simulink model "Aerosonde_modeling_3DOF"  (R2023b)
settings: Solver=VariableStepAuto  StartTime=0.0  StopTime=100  RelTol=1e-3
InitFcn:
  | aerosonde_param
model workspace (MAT data in the model file):
  op_trim1 = opcond.OperatingReport
  op_trim1.Outputs_ = opcond.OutputReport
  op_trim1.Outputs_.yspec_ = 23
  op_trim1.Outputs_.Block_ = 'Aerosonde_modeling_3DOF/Va'
  op_trim1.Outputs_.PortWidth_ = 1
  op_trim1.Outputs_.PortNumber_ = NaN
  op_trim1.Outputs_.y_ = 23
  op_trim1.Outputs_.Known_ = 1
  op_trim1.Outputs_.Min_ = -Inf
  op_trim1.Outputs_.Max_ = Inf
  op_trim1.TerminationString_ = 'Operating point specifications were successfully met.'
  op_trim1.OptimizationOutput_.iterations = 4
  op_trim1.OptimizationOutput_.funcCount = 49
  op_trim1.OptimizationOutput_.lssteplength = 1
  op_trim1.OptimizationOutput_.stepsize = 1.08339920389e-06
  op_trim1.OptimizationOutput_.algorithm = 'active-set'
  op_trim1.OptimizationOutput_.firstorderopt = 6.92917038473e-07
  op_trim1.OptimizationOutput_.constrviolation = 4.1486832541e-10
  op_trim1.OptimizationOutput_.message = 'Local minimum found that satisfies the constraints.
    | 
    | Optimization completed because the objective function is non-decreasing in 
    | feasible directions, to within the value of the optimality tolerance,
    | and constraints are satisfied to within the  value of the constraint tolerance.
    | 
    | <stopping criteria details>
    | 
    | Optimization completed: The first-order optimality measure, 6.929170e-07, is less
    | than options.OptimalityTolerance = 1.000000e-06, and the maximum constraint violation,
    | 4.148683e-10,is less than options.ConstraintTolerance = 1.000000e-06.'
  op_trim1.OptimizationOutput_.bestfeasible.x = [22.8390288243; 2.71638774139; 3.14319268182e-07; -200.000000001; -2.24898193262e-22; 0.11838011473; -0.136728887195; 0.391911265794]
  op_trim1.OptimizationOutput_.bestfeasible.fval = 0
  op_trim1.OptimizationOutput_.bestfeasible.constrviolation = 4.1486832541e-10
  op_trim1.OptimizationOutput_.bestfeasible.firstorderopt = 6.92917038473e-07
  op_trim1.OptimizationOutput_.progress = {'<font face="monospaced"; size=3><BR>', 'Optimizing to solve for all desired dx/dt=0, x(k+1)-x(k)=0, and y=ydes.<BR>', ' <BR>', '(Maximum Error)  Block<BR>', ' ---------------------------------------------------------<BR>', '(6.14386e+00) Aerosonde_modeling_3DOF/3dof (Body Axes)<BR>', '(7.32692e-01) Aerosonde_modeling_3DOF/3dof (Body Axes)<BR>', '(7.37961e-04) Aerosonde_modeling_3DOF/3dof (Body Axes)<BR>', '(2.36211e-06) Aerosonde_modeling_3DOF/3dof (Body Axes)<BR>', '(4.14856e-10) Aerosonde_modeling_3DOF/3dof (Body Axes)<BR>', '(4.14856e-10) Aerosonde_modeling_3DOF/3dof (Body Axes)<BR>', ' <BR>', 'Operating point specifications were successfully met.<BR>'}
  op_trim1.Model_ = 'Aerosonde_modeling_3DOF'
  op_trim1.States_(1) = opcond.StateReport
  op_trim1.States_(1).dx_ = 6.55270405843e-11
  op_trim1.States_(1).Nx_ = 1
  op_trim1.States_(1).Block_ = 'Aerosonde_modeling_3DOF/3dof (Body Axes)'
  op_trim1.States_(1).StateName_ = 'u'
  op_trim1.States_(1).x_ = 22.8390288243
  op_trim1.States_(1).SteadyState_ = 1
  op_trim1.States_(1).dxMin_ = -Inf
  op_trim1.States_(1).dxMax_ = Inf
  op_trim1.States_(1).Known_ = 0
  op_trim1.States_(1).Min_ = -Inf
  op_trim1.States_(1).Max_ = Inf
  op_trim1.States_(2) = opcond.StateReport
  op_trim1.States_(2).dx_ = -4.14855902722e-10
  op_trim1.States_(2).Nx_ = 1
  op_trim1.States_(2).Block_ = 'Aerosonde_modeling_3DOF/3dof (Body Axes)'
  op_trim1.States_(2).StateName_ = 'w'
  op_trim1.States_(2).x_ = 2.71638774139
  op_trim1.States_(2).SteadyState_ = 1
  op_trim1.States_(2).dxMin_ = -Inf
  op_trim1.States_(2).dxMax_ = Inf
  op_trim1.States_(2).Known_ = 0
  op_trim1.States_(2).Min_ = -Inf
  op_trim1.States_(2).Max_ = Inf
  op_trim1.States_(3) = opcond.StateReport
  op_trim1.States_(3).dx_ = 23
  op_trim1.States_(3).Nx_ = 1
  op_trim1.States_(3).Block_ = 'Aerosonde_modeling_3DOF/3dof (Body Axes)'
  op_trim1.States_(3).StateName_ = 'Xe'
  op_trim1.States_(3).x_ = 3.14319268182e-07
  op_trim1.States_(3).SteadyState_ = 0
  op_trim1.States_(3).dxMin_ = -Inf
  op_trim1.States_(3).dxMax_ = Inf
  op_trim1.States_(3).Known_ = 0
  op_trim1.States_(3).Min_ = -Inf
  op_trim1.States_(3).Max_ = Inf
  op_trim1.States_(4) = opcond.StateReport
  op_trim1.States_(4).dx_ = 8.881784197e-16
  op_trim1.States_(4).Nx_ = 1
  op_trim1.States_(4).Block_ = 'Aerosonde_modeling_3DOF/3dof (Body Axes)'
  op_trim1.States_(4).StateName_ = 'Ze'
  op_trim1.States_(4).x_ = -200.000000001
  op_trim1.States_(4).SteadyState_ = 1
  op_trim1.States_(4).dxMin_ = -Inf
  op_trim1.States_(4).dxMax_ = Inf
  op_trim1.States_(4).Known_ = 0
  op_trim1.States_(4).Min_ = -Inf
  op_trim1.States_(4).Max_ = Inf
  op_trim1.States_(5) = opcond.StateReport
  op_trim1.States_(5).dx_ = -1.36577515895e-14
  op_trim1.States_(5).Nx_ = 1
  op_trim1.States_(5).Block_ = 'Aerosonde_modeling_3DOF/3dof (Body Axes)'
  op_trim1.States_(5).StateName_ = 'q'
  op_trim1.States_(5).x_ = -2.24898193262e-22
  op_trim1.States_(5).SteadyState_ = 1
  op_trim1.States_(5).dxMin_ = -Inf
  op_trim1.States_(5).dxMax_ = Inf
  op_trim1.States_(5).Known_ = 0
  op_trim1.States_(5).Min_ = -Inf
  op_trim1.States_(5).Max_ = Inf
  op_trim1.States_(6) = opcond.StateReport
  op_trim1.States_(6).dx_ = -2.24898193262e-22
  op_trim1.States_(6).Nx_ = 1
  op_trim1.States_(6).Block_ = 'Aerosonde_modeling_3DOF/3dof (Body Axes)'
  op_trim1.States_(6).StateName_ = 'theta'
  op_trim1.States_(6).x_ = 0.11838011473
  op_trim1.States_(6).SteadyState_ = 1
  op_trim1.States_(6).dxMin_ = -Inf
  op_trim1.States_(6).dxMax_ = Inf
  op_trim1.States_(6).Known_ = 0
  op_trim1.States_(6).Min_ = -Inf
  op_trim1.States_(6).Max_ = Inf
  op_trim1.Inputs_(1) = opcond.InputReport
  op_trim1.Inputs_(1).Block_ = 'Aerosonde_modeling_3DOF/ELE'
  op_trim1.Inputs_(1).PortWidth_ = 1
  op_trim1.Inputs_(1).PortDimensions_ = [1 1]
  op_trim1.Inputs_(1).u_ = -0.136728887195
  op_trim1.Inputs_(1).Known_ = 0
  op_trim1.Inputs_(1).Min_ = -Inf
  op_trim1.Inputs_(1).Max_ = Inf
  op_trim1.Inputs_(2) = opcond.InputReport
  op_trim1.Inputs_(2).Block_ = 'Aerosonde_modeling_3DOF/THR'
  op_trim1.Inputs_(2).PortWidth_ = 1
  op_trim1.Inputs_(2).PortDimensions_ = [1 1]
  op_trim1.Inputs_(2).u_ = 0.391911265794
  op_trim1.Inputs_(2).Known_ = 0
  op_trim1.Inputs_(2).Min_ = 0
  op_trim1.Inputs_(2).Max_ = 1
  op_trim2 = opcond.OperatingReport
  op_trim2.Outputs_ = opcond.OutputReport
  op_trim2.Outputs_.yspec_ = 23
  op_trim2.Outputs_.Block_ = 'Aerosonde_modeling/Va'
  op_trim2.Outputs_.PortWidth_ = 1
  op_trim2.Outputs_.PortNumber_ = NaN
  op_trim2.Outputs_.y_ = 0.022563556599
  op_trim2.Outputs_.Known_ = 1
  op_trim2.Outputs_.Min_ = -Inf
  op_trim2.Outputs_.Max_ = Inf
  op_trim2.TerminationString_ = 'Operating point specifications were successfully met.'
  op_trim2.OptimizationOutput_.iterations = 1
  op_trim2.OptimizationOutput_.funcCount = 10
  op_trim2.OptimizationOutput_.stepsize = 25.3486722495
  op_trim2.OptimizationOutput_.cgiterations = []
  op_trim2.OptimizationOutput_.firstorderopt = 45.6856066461
  op_trim2.OptimizationOutput_.algorithm = 'levenberg-marquardt'
  op_trim2.OptimizationOutput_.message = 'Local minimum possible.
    | lsqnonlin stopped because the relative size of the current step is less than
    | the value of the step size tolerance.
    | 
    | <stopping criteria details>
    | 
    | Optimization stopped because the relative norm of the current step, 2.607750e-07,
    | is less than options.StepTolerance = 1.000000e-06.'
  op_trim2.OptimizationOutput_.bestfeasible = []
  op_trim2.OptimizationOutput_.constrviolation = []
  op_trim2.OptimizationOutput_.progress = {'<font face="monospaced"; size=3><BR>', 'Optimizing to solve for all desired dx/dt=0, x(k+1)-x(k)=0, and y=ydes.<BR>', ' <BR>', '(Maximum Error)  Block<BR>', ' ---------------------------------------------------------<BR>', '(2.29774e+01) Aerosonde_modeling/Va<BR>', '(2.29774e+01) Aerosonde_modeling/Va<BR>', ' <BR>', 'Operating point specifications were successfully met.<BR>'}
  op_trim2.Model_ = 'Aerosonde_modeling'
  op_trim2.States_(1) = opcond.StateReport
  op_trim2.States_(1).dx_ = -11.6769691065
  op_trim2.States_(1).Nx_ = 1
  op_trim2.States_(1).Block_ = 'Aerosonde_modeling/3dof (Body Axes)'
  op_trim2.States_(1).StateName_ = 'u'
  op_trim2.States_(1).x_ = -0.00779019632016
  op_trim2.States_(1).SteadyState_ = 1
  op_trim2.States_(1).dxMin_ = -Inf
  op_trim2.States_(1).dxMax_ = Inf
  op_trim2.States_(1).Known_ = 0
  op_trim2.States_(1).Min_ = -Inf
  op_trim2.States_(1).Max_ = Inf
  op_trim2.States_(2) = opcond.StateReport
  op_trim2.States_(2).dx_ = -15.7183253748
  op_trim2.States_(2).Nx_ = 1
  op_trim2.States_(2).Block_ = 'Aerosonde_modeling/3dof (Body Axes)'
  op_trim2.States_(2).StateName_ = 'w'
  op_trim2.States_(2).x_ = 0.0211760933056
  op_trim2.States_(2).SteadyState_ = 1
  op_trim2.States_(2).dxMin_ = -Inf
  op_trim2.States_(2).dxMax_ = Inf
  op_trim2.States_(2).Known_ = 0
  op_trim2.States_(2).Min_ = -Inf
  op_trim2.States_(2).Max_ = Inf
  op_trim2.States_(3) = opcond.StateReport
  op_trim2.States_(3).dx_ = 0.0188976239913
  op_trim2.States_(3).Nx_ = 1
  op_trim2.States_(3).Block_ = 'Aerosonde_modeling/3dof (Body Axes)'
  op_trim2.States_(3).StateName_ = 'Xe'
  op_trim2.States_(3).x_ = -7461695.80517
  op_trim2.States_(3).SteadyState_ = 0
  op_trim2.States_(3).dxMin_ = -Inf
  op_trim2.States_(3).dxMax_ = Inf
  op_trim2.States_(3).Known_ = 0
  op_trim2.States_(3).Min_ = -Inf
  op_trim2.States_(3).Max_ = Inf
  op_trim2.States_(4) = opcond.StateReport
  op_trim2.States_(4).dx_ = -0.0123285803676
  op_trim2.States_(4).Nx_ = 1
  op_trim2.States_(4).Block_ = 'Aerosonde_modeling/3dof (Body Axes)'
  op_trim2.States_(4).StateName_ = 'Ze'
  op_trim2.States_(4).x_ = 96918353.295
  op_trim2.States_(4).SteadyState_ = 0
  op_trim2.States_(4).dxMin_ = -Inf
  op_trim2.States_(4).dxMax_ = Inf
  op_trim2.States_(4).Known_ = 0
  op_trim2.States_(4).Min_ = -Inf
  op_trim2.States_(4).Max_ = Inf
  op_trim2.States_(5) = opcond.StateReport
  op_trim2.States_(5).dx_ = -0.000422280268139
  op_trim2.States_(5).Nx_ = 1
  op_trim2.States_(5).Block_ = 'Aerosonde_modeling/3dof (Body Axes)'
  op_trim2.States_(5).StateName_ = 'q'
  op_trim2.States_(5).x_ = -2.06010862536
  op_trim2.States_(5).SteadyState_ = 1
  op_trim2.States_(5).dxMin_ = -Inf
  op_trim2.States_(5).dxMax_ = Inf
  op_trim2.States_(5).Known_ = 0
  op_trim2.States_(5).Min_ = -Inf
  op_trim2.States_(5).Max_ = Inf
  op_trim2.States_(6) = opcond.StateReport
  op_trim2.States_(6).dx_ = -2.06010862536
  op_trim2.States_(6).Nx_ = 1
  op_trim2.States_(6).Block_ = 'Aerosonde_modeling/3dof (Body Axes)'
  op_trim2.States_(6).StateName_ = 'theta'
  op_trim2.States_(6).x_ = 2.50135956362
  op_trim2.States_(6).SteadyState_ = 1
  op_trim2.States_(6).dxMin_ = -Inf
  op_trim2.States_(6).dxMax_ = Inf
  op_trim2.States_(6).Known_ = 0
  op_trim2.States_(6).Min_ = -Inf
  op_trim2.States_(6).Max_ = Inf
  op_trim2.Inputs_(1) = opcond.InputReport
  op_trim2.Inputs_(1).Block_ = 'Aerosonde_modeling/ele'
  op_trim2.Inputs_(1).PortWidth_ = 1
  op_trim2.Inputs_(1).PortDimensions_ = [1 1]
  op_trim2.Inputs_(1).u_ = 6.80738411077e-06
  op_trim2.Inputs_(1).Known_ = 0
  op_trim2.Inputs_(1).Min_ = -Inf
  op_trim2.Inputs_(1).Max_ = Inf
  op_trim2.Inputs_(2) = opcond.InputReport
  op_trim2.Inputs_(2).Block_ = 'Aerosonde_modeling/THR'
  op_trim2.Inputs_(2).PortWidth_ = 1
  op_trim2.Inputs_(2).PortDimensions_ = [1 1]
  op_trim2.Inputs_(2).Known_ = 0
  op_trim2.Inputs_(2).Min_ = 0
  op_trim2.Inputs_(2).Max_ = 1
  op_trim5 = opcond.OperatingReport
  op_trim5.Outputs_ = opcond.OutputReport
  op_trim5.Outputs_.yspec_ = [0; 0; 0; 0; 0; 0; 0]
  op_trim5.Outputs_.Block_ = 'Aerosonde_modeling/States'
  op_trim5.Outputs_.PortWidth_ = 7
  op_trim5.Outputs_.PortNumber_ = NaN
  op_trim5.Outputs_.y_ = [-0.614028193896; 9.4193417265e-05; 2.52756048863; -208278.082793; -1.81540582654e-06; -7461695.80517; 96918353.295]
  op_trim5.Outputs_.Known_ = [0; 0; 0; 0; 0; 0; 0]
  op_trim5.Outputs_.Min_ = [-Inf; -Inf; -Inf; -Inf; -Inf; -Inf; -Inf]
  op_trim5.Outputs_.Max_ = [Inf; Inf; Inf; Inf; Inf; Inf; Inf]
  op_trim5.TerminationString_ = 'Maximum number of function evaluations or iterations was exceeded.  Restart using this resulting solution or use the Optimization Options to increase the number of iterations or function evaluations.'
  op_trim5.OptimizationOutput_.iterations = 101
  op_trim5.OptimizationOutput_.funcCount = 2007
  op_trim5.OptimizationOutput_.lssteplength = 1
  op_trim5.OptimizationOutput_.stepsize = 136552843.933
  op_trim5.OptimizationOutput_.algorithm = 'active-set'
  op_trim5.OptimizationOutput_.firstorderopt = 3.30032720888e+32
  op_trim5.OptimizationOutput_.constrviolation = 15.4518372632
  op_trim5.OptimizationOutput_.message = 'Solver stopped prematurely.
    | 
    | fmincon stopped because it exceeded the function evaluation limit,
    | options.MaxFunctionEvaluations = 2.000000e+03.'
  op_trim5.OptimizationOutput_.bestfeasible = []
  op_trim5.OptimizationOutput_.progress{1} = '<font face="monospaced"; size=3><BR>'
  op_trim5.OptimizationOutput_.progress{2} = 'Optimizing to solve for all desired dx/dt=0, x(k+1)-x(k)=0, and y=ydes.<BR>'
  op_trim5.OptimizationOutput_.progress{3} = ' <BR>'
  op_trim5.OptimizationOutput_.progress{4} = '(Maximum Error)  Block<BR>'
  op_trim5.OptimizationOutput_.progress{5} = ' ---------------------------------------------------------<BR>'
  op_trim5.OptimizationOutput_.progress{6} = '(1.59239e+01) Aerosonde_modeling/3dof (Body Axes)<BR>'
  op_trim5.OptimizationOutput_.progress{7} = '(1.21166e+01) Aerosonde_modeling/3dof (Body Axes)<BR>'
  op_trim5.OptimizationOutput_.progress{8} = '(1.38079e+01) Aerosonde_modeling/3dof (Body Axes)<BR>'
  op_trim5.OptimizationOutput_.progress{9} = '(1.13106e+01) Aerosonde_modeling/3dof (Body Axes)<BR>'
  op_trim5.OptimizationOutput_.progress{10} = '(1.02919e+01) Aerosonde_modeling/3dof (Body Axes)<BR>'
  op_trim5.OptimizationOutput_.progress{11} = '(1.01299e+01) Aerosonde_modeling/3dof (Body Axes)<BR>'
  op_trim5.OptimizationOutput_.progress{12} = '(9.17454e+00) Aerosonde_modeling/3dof (Body Axes)<BR>'
  op_trim5.OptimizationOutput_.progress{13} = '(9.40157e+00) Aerosonde_modeling/3dof (Body Axes)<BR>'
  op_trim5.OptimizationOutput_.progress{14} = '(9.38043e+00) Aerosonde_modeling/3dof (Body Axes)<BR>'
  op_trim5.OptimizationOutput_.progress{15} = '(2.10526e+01) Aerosonde_modeling/3dof (Body Axes)<BR>'
  op_trim5.OptimizationOutput_.progress{16} = '(3.47072e+00) Aerosonde_modeling/3dof (Body Axes)<BR>'
  op_trim5.OptimizationOutput_.progress{17} = '(3.78939e+00) Aerosonde_modeling/3dof (Body Axes)<BR>'
  op_trim5.OptimizationOutput_.progress{18} = '(3.98713e+00) Aerosonde_modeling/3dof (Body Axes)<BR>'
  op_trim5.OptimizationOutput_.progress{19} = '(4.10860e+00) Aerosonde_modeling/3dof (Body Axes)<BR>'
  op_trim5.OptimizationOutput_.progress{20} = '(4.18159e+00) Aerosonde_modeling/3dof (Body Axes)<BR>'
  op_trim5.OptimizationOutput_.progress{21} = '(4.22397e+00) Aerosonde_modeling/3dof (Body Axes)<BR>'
  op_trim5.OptimizationOutput_.progress{22} = '(4.24743e+00) Aerosonde_modeling/3dof (Body Axes)<BR>'
  op_trim5.OptimizationOutput_.progress{23} = '(4.25987e+00) Aerosonde_modeling/3dof (Body Axes)<BR>'
  op_trim5.OptimizationOutput_.progress{24} = '(4.26683e+00) Aerosonde_modeling/3dof (Body Axes)<BR>'
  op_trim5.OptimizationOutput_.progress{25} = '(4.27250e+00) Aerosonde_modeling/3dof (Body Axes)<BR>'
  op_trim5.OptimizationOutput_.progress{26} = '(4.28040e+00) Aerosonde_modeling/3dof (Body Axes)<BR>'
  op_trim5.OptimizationOutput_.progress{27} = '(4.01629e+00) Aerosonde_modeling/3dof (Body Axes)<BR>'
  op_trim5.OptimizationOutput_.progress{28} = '(3.78539e+00) Aerosonde_modeling/3dof (Body Axes)<BR>'
  op_trim5.OptimizationOutput_.progress{29} = '(3.57876e+00) Aerosonde_modeling/3dof (Body Axes)<BR>'
  op_trim5.OptimizationOutput_.progress{30} = '(3.39552e+00) Aerosonde_modeling/3dof (Body Axes)<BR>'
  op_trim5.OptimizationOutput_.progress{31} = '(3.22558e+00) Aerosonde_modeling/3dof (Body Axes)<BR>'
  op_trim5.OptimizationOutput_.progress{32} = '(3.03135e+00) Aerosonde_modeling/3dof (Body Axes)<BR>'
  op_trim5.OptimizationOutput_.progress{33} = '(2.87139e+00) Aerosonde_modeling/3dof (Body Axes)<BR>'
  op_trim5.OptimizationOutput_.progress{34} = '(2.84211e+00) Aerosonde_modeling/3dof (Body Axes)<BR>'
  op_trim5.OptimizationOutput_.progress{35} = '(2.82876e+00) Aerosonde_modeling/3dof (Body Axes)<BR>'
  op_trim5.OptimizationOutput_.progress{36} = '(2.90329e+00) Aerosonde_modeling/3dof (Body Axes)<BR>'
  op_trim5.OptimizationOutput_.progress{37} = '(2.90505e+00) Aerosonde_modeling/3dof (Body Axes)<BR>'
  op_trim5.OptimizationOutput_.progress{38} = '(2.90504e+00) Aerosonde_modeling/3dof (Body Axes)<BR>'
  op_trim5.OptimizationOutput_.progress{39} = '(2.90550e+00) Aerosonde_modeling/3dof (Body Axes)<BR>'
  op_trim5.OptimizationOutput_.progress{40} = '(2.90559e+00) Aerosonde_modeling/3dof (Body Axes)<BR>'
  op_trim5.OptimizationOutput_.progress{41} = '(2.90559e+00) Aerosonde_modeling/3dof (Body Axes)<BR>'
  op_trim5.OptimizationOutput_.progress{42} = '(2.90564e+00) Aerosonde_modeling/3dof (Body Axes)<BR>'
  op_trim5.OptimizationOutput_.progress{43} = '(2.90590e+00) Aerosonde_modeling/3dof (Body Axes)<BR>'
  op_trim5.OptimizationOutput_.progress{44} = '(2.90602e+00) Aerosonde_modeling/3dof (Body Axes)<BR>'
  op_trim5.OptimizationOutput_.progress{45} = '(2.90602e+00) Aerosonde_modeling/3dof (Body Axes)<BR>'
  op_trim5.OptimizationOutput_.progress{46} = '(2.90602e+00) Aerosonde_modeling/3dof (Body Axes)<BR>'
  op_trim5.OptimizationOutput_.progress{47} = '(2.90602e+00) Aerosonde_modeling/3dof (Body Axes)<BR>'
  op_trim5.OptimizationOutput_.progress{48} = '(2.90602e+00) Aerosonde_modeling/3dof (Body Axes)<BR>'
  op_trim5.OptimizationOutput_.progress{49} = '(2.90602e+00) Aerosonde_modeling/3dof (Body Axes)<BR>'
  op_trim5.OptimizationOutput_.progress{50} = '(2.90602e+00) Aerosonde_modeling/3dof (Body Axes)<BR>'
  op_trim5.OptimizationOutput_.progress{51} = '(2.90602e+00) Aerosonde_modeling/3dof (Body Axes)<BR>'
  op_trim5.OptimizationOutput_.progress{52} = '(2.90602e+00) Aerosonde_modeling/3dof (Body Axes)<BR>'
  op_trim5.OptimizationOutput_.progress{53} = '(2.90602e+00) Aerosonde_modeling/3dof (Body Axes)<BR>'
  op_trim5.OptimizationOutput_.progress{54} = '(2.90602e+00) Aerosonde_modeling/3dof (Body Axes)<BR>'
  op_trim5.OptimizationOutput_.progress{55} = '(2.90602e+00) Aerosonde_modeling/3dof (Body Axes)<BR>'
  op_trim5.OptimizationOutput_.progress{56} = '(2.90602e+00) Aerosonde_modeling/3dof (Body Axes)<BR>'
  op_trim5.OptimizationOutput_.progress{57} = '(2.90602e+00) Aerosonde_modeling/3dof (Body Axes)<BR>'
  op_trim5.OptimizationOutput_.progress{58} = '(2.90602e+00) Aerosonde_modeling/3dof (Body Axes)<BR>'
  op_trim5.OptimizationOutput_.progress{59} = '(2.90602e+00) Aerosonde_modeling/3dof (Body Axes)<BR>'
  op_trim5.OptimizationOutput_.progress{60} = '(2.90602e+00) Aerosonde_modeling/3dof (Body Axes)<BR>'
  op_trim5.OptimizationOutput_.progress{61} = '(2.90602e+00) Aerosonde_modeling/3dof (Body Axes)<BR>'
  op_trim5.OptimizationOutput_.progress{62} = '(2.90602e+00) Aerosonde_modeling/3dof (Body Axes)<BR>'
  op_trim5.OptimizationOutput_.progress{63} = '(2.90602e+00) Aerosonde_modeling/3dof (Body Axes)<BR>'
  op_trim5.OptimizationOutput_.progress{64} = '(2.90602e+00) Aerosonde_modeling/3dof (Body Axes)<BR>'
  op_trim5.OptimizationOutput_.progress{65} = '(2.90602e+00) Aerosonde_modeling/3dof (Body Axes)<BR>'
  op_trim5.OptimizationOutput_.progress{66} = '(2.90602e+00) Aerosonde_modeling/3dof (Body Axes)<BR>'
  op_trim5.OptimizationOutput_.progress{67} = '(2.90602e+00) Aerosonde_modeling/3dof (Body Axes)<BR>'
  op_trim5.OptimizationOutput_.progress{68} = '(2.90602e+00) Aerosonde_modeling/3dof (Body Axes)<BR>'
  op_trim5.OptimizationOutput_.progress{69} = '(2.90602e+00) Aerosonde_modeling/3dof (Body Axes)<BR>'
  op_trim5.OptimizationOutput_.progress{70} = '(2.90602e+00) Aerosonde_modeling/3dof (Body Axes)<BR>'
  op_trim5.OptimizationOutput_.progress{71} = '(2.90602e+00) Aerosonde_modeling/3dof (Body Axes)<BR>'
  op_trim5.OptimizationOutput_.progress{72} = '(2.90606e+00) Aerosonde_modeling/3dof (Body Axes)<BR>'
  op_trim5.OptimizationOutput_.progress{73} = '(2.75093e+00) Aerosonde_modeling/3dof (Body Axes)<BR>'
  op_trim5.OptimizationOutput_.progress{74} = '(3.54582e+00) Aerosonde_modeling/3dof (Body Axes)<BR>'
  op_trim5.OptimizationOutput_.progress{75} = '(3.89297e+00) Aerosonde_modeling/3dof (Body Axes)<BR>'
  op_trim5.OptimizationOutput_.progress{76} = '(4.14986e+00) Aerosonde_modeling/3dof (Body Axes)<BR>'
  op_trim5.OptimizationOutput_.progress{77} = '(3.55999e+00) Aerosonde_modeling/3dof (Body Axes)<BR>'
  op_trim5.OptimizationOutput_.progress{78} = '(3.20494e+00) Aerosonde_modeling/3dof (Body Axes)<BR>'
  op_trim5.OptimizationOutput_.progress{79} = '(3.18668e+00) Aerosonde_modeling/3dof (Body Axes)<BR>'
  op_trim5.OptimizationOutput_.progress{80} = '(3.13765e+00) Aerosonde_modeling/3dof (Body Axes)<BR>'
  op_trim5.OptimizationOutput_.progress{81} = '(2.68545e+00) Aerosonde_modeling/3dof (Body Axes)<BR>'
  op_trim5.OptimizationOutput_.progress{82} = '(1.76493e-01) Aerosonde_modeling/3dof (Body Axes)<BR>'
  op_trim5.OptimizationOutput_.progress{83} = '(2.34829e-01) Aerosonde_modeling/3dof (Body Axes)<BR>'
  op_trim5.OptimizationOutput_.progress{84} = '(2.35613e-01) Aerosonde_modeling/3dof (Body Axes)<BR>'
  op_trim5.OptimizationOutput_.progress{85} = '(2.35160e-01) Aerosonde_modeling/3dof (Body Axes)<BR>'
  op_trim5.OptimizationOutput_.progress{86} = '(2.34644e-01) Aerosonde_modeling/3dof (Body Axes)<BR>'
  op_trim5.OptimizationOutput_.progress{87} = '(2.34133e-01) Aerosonde_modeling/3dof (Body Axes)<BR>'
  op_trim5.OptimizationOutput_.progress{88} = '(2.33579e-01) Aerosonde_modeling/3dof (Body Axes)<BR>'
  op_trim5.OptimizationOutput_.progress{89} = '(2.33121e-01) Aerosonde_modeling/3dof (Body Axes)<BR>'
  op_trim5.OptimizationOutput_.progress{90} = '(2.33001e-01) Aerosonde_modeling/3dof (Body Axes)<BR>'
  op_trim5.OptimizationOutput_.progress{91} = '(2.32485e-01) Aerosonde_modeling/3dof (Body Axes)<BR>'
  op_trim5.OptimizationOutput_.progress{92} = '(2.31943e-01) Aerosonde_modeling/3dof (Body Axes)<BR>'
  op_trim5.OptimizationOutput_.progress{93} = '(2.31688e-01) Aerosonde_modeling/3dof (Body Axes)<BR>'
  op_trim5.OptimizationOutput_.progress{94} = '(2.31184e-01) Aerosonde_modeling/3dof (Body Axes)<BR>'
  op_trim5.OptimizationOutput_.progress{95} = '(2.30618e-01) Aerosonde_modeling/3dof (Body Axes)<BR>'
  op_trim5.OptimizationOutput_.progress{96} = '(2.44391e-02) Aerosonde_modeling/3dof (Body Axes)<BR>'
  op_trim5.OptimizationOutput_.progress{97} = '(4.66230e-02) Aerosonde_modeling/3dof (Body Axes)<BR>'
  op_trim5.OptimizationOutput_.progress{98} = '(2.92160e-03) Aerosonde_modeling/3dof (Body Axes)<BR>'
  op_trim5.OptimizationOutput_.progress{99} = '(1.24310e-03) Aerosonde_modeling/3dof (Body Axes)<BR>'
  op_trim5.OptimizationOutput_.progress{100} = '(1.24307e-03) Aerosonde_modeling/3dof (Body Axes)<BR>'
  op_trim5.OptimizationOutput_.progress{101} = '(1.24305e-03) Aerosonde_modeling/3dof (Body Axes)<BR>'
  op_trim5.OptimizationOutput_.progress{102} = '(1.24303e-03) Aerosonde_modeling/3dof (Body Axes)<BR>'
  op_trim5.OptimizationOutput_.progress{103} = '(1.24300e-03) Aerosonde_modeling/3dof (Body Axes)<BR>'
  op_trim5.OptimizationOutput_.progress{104} = '(1.24298e-03) Aerosonde_modeling/3dof (Body Axes)<BR>'
  op_trim5.OptimizationOutput_.progress{105} = '(1.24296e-03) Aerosonde_modeling/3dof (Body Axes)<BR>'
  op_trim5.OptimizationOutput_.progress{106} = '(1.24293e-03) Aerosonde_modeling/3dof (Body Axes)<BR>'
  op_trim5.OptimizationOutput_.progress{107} = '(1.54518e+01) Aerosonde_modeling/3dof (Body Axes)<BR>'
  op_trim5.OptimizationOutput_.progress{108} = '(1.24293e-03) Aerosonde_modeling/3dof (Body Axes)<BR>'
  op_trim5.OptimizationOutput_.progress{109} = ' <BR>'
  op_trim5.OptimizationOutput_.progress{110} = 'Maximum number of function evaluations or iterations was exceeded.  Restart using this resulting solution or use the Optimization Options to increase the number of iterations or function evaluations.<BR>'
  op_trim5.Model_ = 'Aerosonde_modeling'
  op_trim5.States_(1) = opcond.StateReport
  op_trim5.States_(1).dx_ = -0.00097150794859
  op_trim5.States_(1).Nx_ = 1
  op_trim5.States_(1).Block_ = 'Aerosonde_modeling/3dof (Body Axes)'
  op_trim5.States_(1).StateName_ = 'u'
  op_trim5.States_(1).x_ = -7.69874592357e-05
  op_trim5.States_(1).SteadyState_ = 1
  op_trim5.States_(1).dxMin_ = -Inf
  op_trim5.States_(1).dxMax_ = Inf
  op_trim5.States_(1).Known_ = 0
  op_trim5.States_(1).Min_ = -Inf
  op_trim5.States_(1).Max_ = Inf
  op_trim5.States_(2) = opcond.StateReport
  op_trim5.States_(2).dx_ = -0.00124293328653
  op_trim5.States_(2).Nx_ = 1
  op_trim5.States_(2).Block_ = 'Aerosonde_modeling/3dof (Body Axes)'
  op_trim5.States_(2).StateName_ = 'w'
  op_trim5.States_(2).x_ = 5.42709035901e-05
  op_trim5.States_(2).SteadyState_ = 1
  op_trim5.States_(2).dxMin_ = -Inf
  op_trim5.States_(2).dxMax_ = Inf
  op_trim5.States_(2).Known_ = 0
  op_trim5.States_(2).Min_ = -Inf
  op_trim5.States_(2).Max_ = Inf
  op_trim5.States_(3) = opcond.StateReport
  op_trim5.States_(3).dx_ = 9.41934172643e-05
  op_trim5.States_(3).Nx_ = 1
  op_trim5.States_(3).Block_ = 'Aerosonde_modeling/3dof (Body Axes)'
  op_trim5.States_(3).StateName_ = 'Xe'
  op_trim5.States_(3).x_ = -7461695.80517
  op_trim5.States_(3).SteadyState_ = 0
  op_trim5.States_(3).dxMin_ = -Inf
  op_trim5.States_(3).dxMax_ = Inf
  op_trim5.States_(3).Known_ = 0
  op_trim5.States_(3).Min_ = -Inf
  op_trim5.States_(3).Max_ = Inf
  op_trim5.States_(4) = opcond.StateReport
  op_trim5.States_(4).dx_ = 3.74047871724e-10
  op_trim5.States_(4).Nx_ = 1
  op_trim5.States_(4).Block_ = 'Aerosonde_modeling/3dof (Body Axes)'
  op_trim5.States_(4).StateName_ = 'Ze'
  op_trim5.States_(4).x_ = 96918353.295
  op_trim5.States_(4).SteadyState_ = 1
  op_trim5.States_(4).dxMin_ = -Inf
  op_trim5.States_(4).dxMax_ = Inf
  op_trim5.States_(4).Known_ = 0
  op_trim5.States_(4).Min_ = -Inf
  op_trim5.States_(4).Max_ = Inf
  op_trim5.States_(5) = opcond.StateReport
  op_trim5.States_(5).dx_ = -1.81540582654e-06
  op_trim5.States_(5).Nx_ = 1
  op_trim5.States_(5).Block_ = 'Aerosonde_modeling/3dof (Body Axes)'
  op_trim5.States_(5).StateName_ = 'q'
  op_trim5.States_(5).x_ = -208278.082793
  op_trim5.States_(5).SteadyState_ = 1
  op_trim5.States_(5).dxMin_ = -Inf
  op_trim5.States_(5).dxMax_ = Inf
  op_trim5.States_(5).Known_ = 0
  op_trim5.States_(5).Min_ = -Inf
  op_trim5.States_(5).Max_ = Inf
  op_trim5.States_(6) = opcond.StateReport
  op_trim5.States_(6).dx_ = -208278.082793
  op_trim5.States_(6).Nx_ = 1
  op_trim5.States_(6).Block_ = 'Aerosonde_modeling/3dof (Body Axes)'
  op_trim5.States_(6).StateName_ = 'theta'
  op_trim5.States_(6).x_ = 2.52756048863
  op_trim5.States_(6).SteadyState_ = 0
  op_trim5.States_(6).dxMin_ = -Inf
  op_trim5.States_(6).dxMax_ = Inf
  op_trim5.States_(6).Known_ = 0
  op_trim5.States_(6).Min_ = -Inf
  op_trim5.States_(6).Max_ = Inf
  op_trim7 = opcond.OperatingReport
  op_trim7.Outputs_ = opcond.OutputReport
  op_trim7.Outputs_.yspec_ = 23
  op_trim7.Outputs_.Block_ = 'Aerosonde_modeling/Va'
  op_trim7.Outputs_.PortWidth_ = 1
  op_trim7.Outputs_.PortNumber_ = NaN
  op_trim7.Outputs_.y_ = 23
  op_trim7.Outputs_.Known_ = 1
  op_trim7.Outputs_.Min_ = -Inf
  op_trim7.Outputs_.Max_ = Inf
  op_trim7.TerminationString_ = 'Operating point specifications were successfully met.'
  op_trim7.OptimizationOutput_.iterations = 7
  op_trim7.OptimizationOutput_.funcCount = 73
  op_trim7.OptimizationOutput_.stepsize = 1.70608835288e-06
  op_trim7.OptimizationOutput_.cgiterations = []
  op_trim7.OptimizationOutput_.firstorderopt = 1.00605215098e-08
  op_trim7.OptimizationOutput_.algorithm = 'levenberg-marquardt'
  op_trim7.OptimizationOutput_.message = 'Local minimum found.
    | 
    | Optimization completed because the size of the gradient is less than
    | 1e-4 times the value of the function tolerance.
    | 
    | <stopping criteria details>
    | 
    | Optimization completed: The relative first-order optimality measure, 2.739437e-11,
    | is less than 1e-4*options.FunctionTolerance = 1.000000e-10.'
  op_trim7.OptimizationOutput_.bestfeasible = []
  op_trim7.OptimizationOutput_.constrviolation = []
  op_trim7.OptimizationOutput_.progress = {'<font face="monospaced"; size=3><BR>', 'Optimizing to solve for all desired dx/dt=0, x(k+1)-x(k)=0, and y=ydes.<BR>', ' <BR>', '(Maximum Error)  Block<BR>', ' ---------------------------------------------------------<BR>', '(1.59539e+01) Aerosonde_modeling/3dof (Body Axes)<BR>', '(5.98669e-01) Aerosonde_modeling/3dof (Body Axes)<BR>', '(3.18893e-01) Aerosonde_modeling/3dof (Body Axes)<BR>', '(2.40139e-01) Aerosonde_modeling/3dof (Body Axes)<BR>', '(2.06886e-01) Aerosonde_modeling/3dof (Body Axes)<BR>', '(2.80263e-03) Aerosonde_modeling/3dof (Body Axes)<BR>', '(3.16724e-07) Aerosonde_modeling/3dof (Body Axes)<BR>', '(4.32534e-09) Aerosonde_modeling/3dof (Body Axes)<BR>', '(4.32534e-09) Aerosonde_modeling/3dof (Body Axes)<BR>', ' <BR>', 'Operating point specifications were successfully met.<BR>'}
  op_trim7.Model_ = 'Aerosonde_modeling'
  op_trim7.States_(1) = opcond.StateReport
  op_trim7.States_(1).dx_ = -1.45716741756e-13
  op_trim7.States_(1).Nx_ = 1
  op_trim7.States_(1).Block_ = 'Aerosonde_modeling/3dof (Body Axes)'
  op_trim7.States_(1).StateName_ = 'u'
  op_trim7.States_(1).x_ = 21.9071658234
  op_trim7.States_(1).SteadyState_ = 1
  op_trim7.States_(1).dxMin_ = -Inf
  op_trim7.States_(1).dxMax_ = Inf
  op_trim7.States_(1).Known_ = 0
  op_trim7.States_(1).Min_ = -Inf
  op_trim7.States_(1).Max_ = Inf
  op_trim7.States_(2) = opcond.StateReport
  op_trim7.States_(2).dx_ = 6.74224343065e-13
  op_trim7.States_(2).Nx_ = 1
  op_trim7.States_(2).Block_ = 'Aerosonde_modeling/3dof (Body Axes)'
  op_trim7.States_(2).StateName_ = 'w'
  op_trim7.States_(2).x_ = 7.0054325768
  op_trim7.States_(2).SteadyState_ = 1
  op_trim7.States_(2).dxMin_ = -Inf
  op_trim7.States_(2).dxMax_ = Inf
  op_trim7.States_(2).Known_ = 0
  op_trim7.States_(2).Min_ = -Inf
  op_trim7.States_(2).Max_ = Inf
  op_trim7.States_(3) = opcond.StateReport
  op_trim7.States_(3).dx_ = 23
  op_trim7.States_(3).Nx_ = 1
  op_trim7.States_(3).Block_ = 'Aerosonde_modeling/3dof (Body Axes)'
  op_trim7.States_(3).StateName_ = 'Xe'
  op_trim7.States_(3).x_ = -1.90575601527e-07
  op_trim7.States_(3).SteadyState_ = 0
  op_trim7.States_(3).dxMin_ = -Inf
  op_trim7.States_(3).dxMax_ = Inf
  op_trim7.States_(3).Known_ = 0
  op_trim7.States_(3).Min_ = -Inf
  op_trim7.States_(3).Max_ = Inf
  op_trim7.States_(4) = opcond.StateReport
  op_trim7.States_(4).dx_ = -7.46069872548e-14
  op_trim7.States_(4).Nx_ = 1
  op_trim7.States_(4).Block_ = 'Aerosonde_modeling/3dof (Body Axes)'
  op_trim7.States_(4).StateName_ = 'Ze'
  op_trim7.States_(4).x_ = -200.000000001
  op_trim7.States_(4).SteadyState_ = 1
  op_trim7.States_(4).dxMin_ = -Inf
  op_trim7.States_(4).dxMax_ = Inf
  op_trim7.States_(4).Known_ = 0
  op_trim7.States_(4).Min_ = -Inf
  op_trim7.States_(4).Max_ = Inf
  op_trim7.States_(5) = opcond.StateReport
  op_trim7.States_(5).dx_ = 4.32533543156e-09
  op_trim7.States_(5).Nx_ = 1
  op_trim7.States_(5).Block_ = 'Aerosonde_modeling/3dof (Body Axes)'
  op_trim7.States_(5).StateName_ = 'q'
  op_trim7.States_(5).x_ = -1.72917137263e-11
  op_trim7.States_(5).SteadyState_ = 1
  op_trim7.States_(5).dxMin_ = -Inf
  op_trim7.States_(5).dxMax_ = Inf
  op_trim7.States_(5).Known_ = 0
  op_trim7.States_(5).Min_ = -Inf
  op_trim7.States_(5).Max_ = Inf
  op_trim7.States_(6) = opcond.StateReport
  op_trim7.States_(6).dx_ = -1.72917137263e-11
  op_trim7.States_(6).Nx_ = 1
  op_trim7.States_(6).Block_ = 'Aerosonde_modeling/3dof (Body Axes)'
  op_trim7.States_(6).StateName_ = 'theta'
  op_trim7.States_(6).x_ = 0.309501673025
  op_trim7.States_(6).SteadyState_ = 1
  op_trim7.States_(6).dxMin_ = -Inf
  op_trim7.States_(6).dxMax_ = Inf
  op_trim7.States_(6).Known_ = 0
  op_trim7.States_(6).Min_ = -Inf
  op_trim7.States_(6).Max_ = Inf
  op_trim7.Inputs_(1) = opcond.InputReport
  op_trim7.Inputs_(1).Block_ = 'Aerosonde_modeling/ELE'
  op_trim7.Inputs_(1).PortWidth_ = 1
  op_trim7.Inputs_(1).PortDimensions_ = [1 1]
  op_trim7.Inputs_(1).u_ = -0.281981271788
  op_trim7.Inputs_(1).Known_ = 0
  op_trim7.Inputs_(1).Min_ = -Inf
  op_trim7.Inputs_(1).Max_ = Inf
  op_trim7.Inputs_(2) = opcond.InputReport
  op_trim7.Inputs_(2).Block_ = 'Aerosonde_modeling/THR'
  op_trim7.Inputs_(2).PortWidth_ = 1
  op_trim7.Inputs_(2).PortDimensions_ = [1 1]
  op_trim7.Inputs_(2).u_ = 0.766164059306
  op_trim7.Inputs_(2).Known_ = 0
  op_trim7.Inputs_(2).Min_ = 0
  op_trim7.Inputs_(2).Max_ = 1
  op_trim8 = opcond.OperatingReport
  op_trim8.Outputs_ = opcond.OutputReport
  op_trim8.Outputs_.yspec_ = 23
  op_trim8.Outputs_.Block_ = 'Aerosonde_modeling/Va'
  op_trim8.Outputs_.PortWidth_ = 1
  op_trim8.Outputs_.PortNumber_ = NaN
  op_trim8.Outputs_.y_ = 23
  op_trim8.Outputs_.Known_ = 1
  op_trim8.Outputs_.Min_ = -Inf
  op_trim8.Outputs_.Max_ = Inf
  op_trim8.TerminationString_ = 'Operating point specifications were successfully met.'
  op_trim8.OptimizationOutput_.iterations = 7
  op_trim8.OptimizationOutput_.funcCount = 73
  op_trim8.OptimizationOutput_.stepsize = 1.70608835288e-06
  op_trim8.OptimizationOutput_.cgiterations = []
  op_trim8.OptimizationOutput_.firstorderopt = 1.00605215098e-08
  op_trim8.OptimizationOutput_.algorithm = 'levenberg-marquardt'
  op_trim8.OptimizationOutput_.message = 'Local minimum found.
    | 
    | Optimization completed because the size of the gradient is less than
    | 1e-4 times the value of the function tolerance.
    | 
    | <stopping criteria details>
    | 
    | Optimization completed: The relative first-order optimality measure, 2.739437e-11,
    | is less than 1e-4*options.FunctionTolerance = 1.000000e-10.'
  op_trim8.OptimizationOutput_.bestfeasible = []
  op_trim8.OptimizationOutput_.constrviolation = []
  op_trim8.OptimizationOutput_.progress = {'<font face="monospaced"; size=3><BR>', 'Optimizing to solve for all desired dx/dt=0, x(k+1)-x(k)=0, and y=ydes.<BR>', ' <BR>', '(Maximum Error)  Block<BR>', ' ---------------------------------------------------------<BR>', '(1.59539e+01) Aerosonde_modeling/3dof (Body Axes)<BR>', '(5.98669e-01) Aerosonde_modeling/3dof (Body Axes)<BR>', '(3.18893e-01) Aerosonde_modeling/3dof (Body Axes)<BR>', '(2.40139e-01) Aerosonde_modeling/3dof (Body Axes)<BR>', '(2.06886e-01) Aerosonde_modeling/3dof (Body Axes)<BR>', '(2.80263e-03) Aerosonde_modeling/3dof (Body Axes)<BR>', '(3.16724e-07) Aerosonde_modeling/3dof (Body Axes)<BR>', '(4.32534e-09) Aerosonde_modeling/3dof (Body Axes)<BR>', '(4.32534e-09) Aerosonde_modeling/3dof (Body Axes)<BR>', ' <BR>', 'Operating point specifications were successfully met.<BR>'}
  op_trim8.Model_ = 'Aerosonde_modeling'
  op_trim8.States_(1) = opcond.StateReport
  op_trim8.States_(1).dx_ = -1.45716741756e-13
  op_trim8.States_(1).Nx_ = 1
  op_trim8.States_(1).Block_ = 'Aerosonde_modeling/3dof (Body Axes)'
  op_trim8.States_(1).StateName_ = 'u'
  op_trim8.States_(1).x_ = 21.9071658234
  op_trim8.States_(1).SteadyState_ = 1
  op_trim8.States_(1).dxMin_ = -Inf
  op_trim8.States_(1).dxMax_ = Inf
  op_trim8.States_(1).Known_ = 0
  op_trim8.States_(1).Min_ = -Inf
  op_trim8.States_(1).Max_ = Inf
  op_trim8.States_(2) = opcond.StateReport
  op_trim8.States_(2).dx_ = 6.74224343065e-13
  op_trim8.States_(2).Nx_ = 1
  op_trim8.States_(2).Block_ = 'Aerosonde_modeling/3dof (Body Axes)'
  op_trim8.States_(2).StateName_ = 'w'
  op_trim8.States_(2).x_ = 7.0054325768
  op_trim8.States_(2).SteadyState_ = 1
  op_trim8.States_(2).dxMin_ = -Inf
  op_trim8.States_(2).dxMax_ = Inf
  op_trim8.States_(2).Known_ = 0
  op_trim8.States_(2).Min_ = -Inf
  op_trim8.States_(2).Max_ = Inf
  op_trim8.States_(3) = opcond.StateReport
  op_trim8.States_(3).dx_ = 23
  op_trim8.States_(3).Nx_ = 1
  op_trim8.States_(3).Block_ = 'Aerosonde_modeling/3dof (Body Axes)'
  op_trim8.States_(3).StateName_ = 'Xe'
  op_trim8.States_(3).x_ = -1.90575601527e-07
  op_trim8.States_(3).SteadyState_ = 0
  op_trim8.States_(3).dxMin_ = -Inf
  op_trim8.States_(3).dxMax_ = Inf
  op_trim8.States_(3).Known_ = 0
  op_trim8.States_(3).Min_ = -Inf
  op_trim8.States_(3).Max_ = Inf
  op_trim8.States_(4) = opcond.StateReport
  op_trim8.States_(4).dx_ = -7.46069872548e-14
  op_trim8.States_(4).Nx_ = 1
  op_trim8.States_(4).Block_ = 'Aerosonde_modeling/3dof (Body Axes)'
  op_trim8.States_(4).StateName_ = 'Ze'
  op_trim8.States_(4).x_ = -200.000000001
  op_trim8.States_(4).SteadyState_ = 1
  op_trim8.States_(4).dxMin_ = -Inf
  op_trim8.States_(4).dxMax_ = Inf
  op_trim8.States_(4).Known_ = 0
  op_trim8.States_(4).Min_ = -Inf
  op_trim8.States_(4).Max_ = Inf
  op_trim8.States_(5) = opcond.StateReport
  op_trim8.States_(5).dx_ = 4.32533543156e-09
  op_trim8.States_(5).Nx_ = 1
  op_trim8.States_(5).Block_ = 'Aerosonde_modeling/3dof (Body Axes)'
  op_trim8.States_(5).StateName_ = 'q'
  op_trim8.States_(5).x_ = -1.72917137263e-11
  op_trim8.States_(5).SteadyState_ = 1
  op_trim8.States_(5).dxMin_ = -Inf
  op_trim8.States_(5).dxMax_ = Inf
  op_trim8.States_(5).Known_ = 0
  op_trim8.States_(5).Min_ = -Inf
  op_trim8.States_(5).Max_ = Inf
  op_trim8.States_(6) = opcond.StateReport
  op_trim8.States_(6).dx_ = -1.72917137263e-11
  op_trim8.States_(6).Nx_ = 1
  op_trim8.States_(6).Block_ = 'Aerosonde_modeling/3dof (Body Axes)'
  op_trim8.States_(6).StateName_ = 'theta'
  op_trim8.States_(6).x_ = 0.309501673025
  op_trim8.States_(6).SteadyState_ = 1
  op_trim8.States_(6).dxMin_ = -Inf
  op_trim8.States_(6).dxMax_ = Inf
  op_trim8.States_(6).Known_ = 0
  op_trim8.States_(6).Min_ = -Inf
  op_trim8.States_(6).Max_ = Inf
  op_trim8.Inputs_(1) = opcond.InputReport
  op_trim8.Inputs_(1).Block_ = 'Aerosonde_modeling/ELE'
  op_trim8.Inputs_(1).PortWidth_ = 1
  op_trim8.Inputs_(1).PortDimensions_ = [1 1]
  op_trim8.Inputs_(1).u_ = -0.281981271788
  op_trim8.Inputs_(1).Known_ = 0
  op_trim8.Inputs_(1).Min_ = -Inf
  op_trim8.Inputs_(1).Max_ = Inf
  op_trim8.Inputs_(2) = opcond.InputReport
  op_trim8.Inputs_(2).Block_ = 'Aerosonde_modeling/THR'
  op_trim8.Inputs_(2).PortWidth_ = 1
  op_trim8.Inputs_(2).PortDimensions_ = [1 1]
  op_trim8.Inputs_(2).u_ = 0.766164059306
  op_trim8.Inputs_(2).Known_ = 0
  op_trim8.Inputs_(2).Min_ = 0
  op_trim8.Inputs_(2).Max_ = 1
values from neighbouring files (symbols this model uses):
  c = 0.18994    [aerosonde_param.m]
  CD_0 = 0.03    [aerosonde_param.m]
  CD_a = 0.30    (= 0.3)    [aerosonde_param.m]
  CD_e = 0    [aerosonde_param.m]
  CD_q = 0    [aerosonde_param.m]
  CL_0 = 0.28    [aerosonde_param.m]
  CL_a = 3.45    [aerosonde_param.m]
  CL_e = -0.36    [aerosonde_param.m]
  CL_q = 0    [aerosonde_param.m]
  CM_0 = -0.02338    [aerosonde_param.m]
  CM_a = -0.38    [aerosonde_param.m]
  CM_e = -0.5    [aerosonde_param.m]
  CM_q = -3.6    [aerosonde_param.m]
  m = 13.5    [aerosonde_param.m]
  S = 0.55    [aerosonde_param.m]
undefined symbols (not defined in the file or in its folder): deg, rad, s
libraries: aerolibconvert2 x2
settings Model: Creator=seungshin  LastModifiedBy=1234
settings DataIOCC: ExternalInput=getinputstruct(op_trim1)  InitialState=getstatestruct(op_trim1)  LoadExternalInput=on  LoadInitialState=on

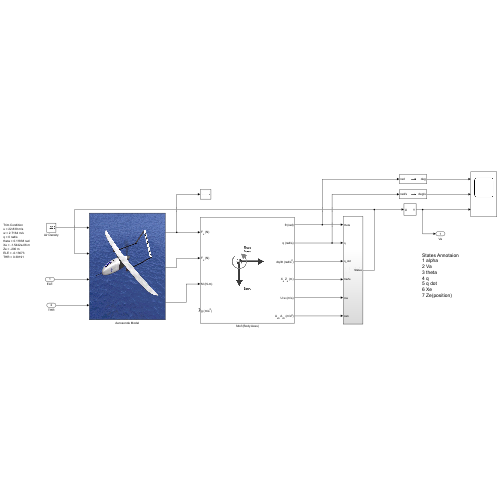
[thumbnail: Simulink's stored preview of the top-level diagram]
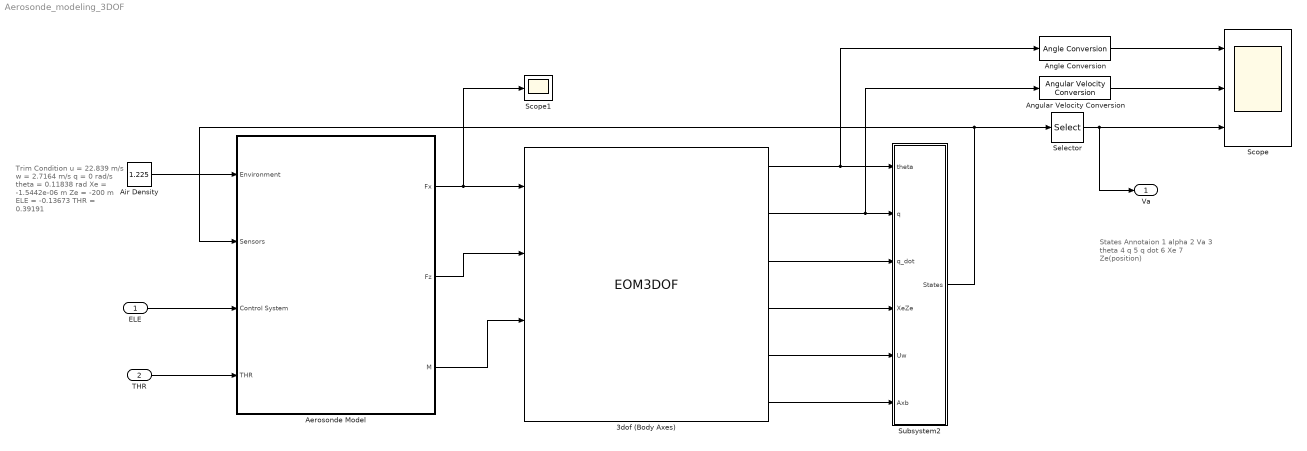
== system Aerosonde_modeling_3DOF ==
  note: Trim Condition
      | u = 22.839 m/s
      | w = 2.7164 m/s
      | q = 0 rad/s
      | theta = 0.11838 rad
      | Xe = -1.5442e-06 m
      | Ze = -200 m
      | ELE = -0.13673
      | THR = 0.39191
  note: States Annotaion
      | 1 alpha
      | 2 Va
      | 3 theta
      | 4 q
      | 5 q dot
      | 6 Xe
      | 7 Ze(position)
  ELE : Inport
  THR : Inport  Port=2
  3dof (Body Axes) : EOM3DOF  v_ini=23  pos_ini=[0 -200]  mass=m  Iyy=Iyy  g_in=External  vel_statename={'u','w'}  pos_statename={'Xe','Ze'}  q_statename='q'  theta_statename='theta'
  Aerosonde Model : Subsystem
      mask Display: image('Aerosonde.jpg');
  Air Density : Constant  Value=1.225
  Angle Conversion : aerolibconvert2/Angle Conversion  IU=rad  OU=deg
  Angular Velocity Conversion : aerolibconvert2/Angular Velocity Conversion  IU=rad/s  OU=deg/s
  Scope : Scope  NumInputPorts=3
  Scope1 : Scope
  Selector : Selector  InputPortWidth=7  IndexOptions=Index vector (dialog)  Indices=[2]  OutputSizes=1
  Subsystem2 : Subsystem
  Va : Outport
  wires:
  3dof (Body Axes)/5 -> Subsystem2/5(Uw)
  3dof (Body Axes)/3 -> Subsystem2/3(q_dot)
  3dof (Body Axes)/4 -> Subsystem2/4(XeZe)
  3dof (Body Axes)/6 -> Subsystem2/6(Axb)
  Subsystem2/1(States) -> Aerosonde Model/2(Sensors), Selector/1
  Aerosonde Model/1(Fx) -> Scope1/1, 3dof (Body Axes)/1
  Aerosonde Model/2(Fz) -> 3dof (Body Axes)/2
  Aerosonde Model/3(M) -> 3dof (Body Axes)/3
  3dof (Body Axes)/2 -> Angular Velocity Conversion/1, Subsystem2/2(q)
  3dof (Body Axes)/1 -> Subsystem2/1(theta), Angle Conversion/1
  Selector/1 -> Scope/3, Va/1
  ELE/1 -> Aerosonde Model/3(Control System)
  THR/1 -> Aerosonde Model/4(THR)
  Angle Conversion/1 -> Scope/1
  Angular Velocity Conversion/1 -> Scope/2
  Air Density/1 -> Aerosonde Model/1(Environment)

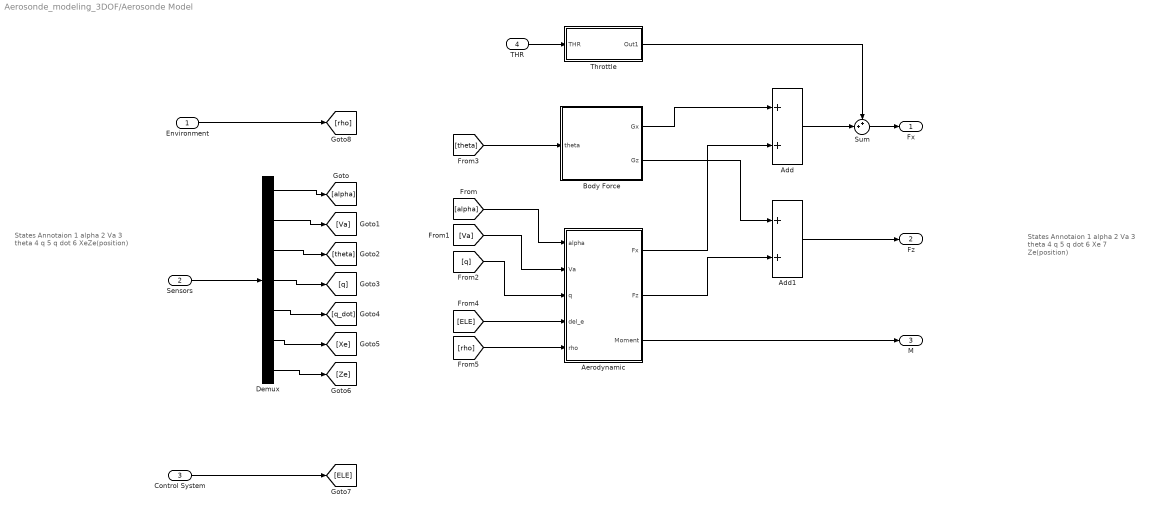
== system Aerosonde_modeling_3DOF/Aerosonde Model ==
  note: States Annotaion
      | 1 alpha
      | 2 Va
      | 3 theta
      | 4 q
      | 5 q dot
      | 6 Xe
      | 7 Ze(position)
  note: States Annotaion
      | 1 alpha
      | 2 Va
      | 3 theta
      | 4 q
      | 5 q dot
      | 6 XeZe(position)
  Environment : Inport
  Sensors : Inport  Port=2
  Control System : Inport  Port=3
  THR : Inport  Port=4
  Add : Sum
  Add1 : Sum
  Aerodynamic : Subsystem
  Body Force : Subsystem
  Demux : Demux  Outputs=7
  Sum : Sum  Inputs=++|
  Throttle : Subsystem
  Fx : Outport
  Fz : Outport  Port=2
  M : Outport  Port=3
  wires:
  [rho] -> Aerodynamic/5(rho)
  Aerodynamic/3(Moment) -> M/1
  [alpha] -> Aerodynamic/1(alpha)
  [Va] -> Aerodynamic/2(Va)
  Sensors/1 -> Demux/1
  Demux/1 -> [alpha]
  Demux/2 -> [Va]
  Demux/3 -> [theta]
  Demux/4 -> [q]
  Demux/5 -> [q_dot]
  Demux/6 -> [Xe]
  [q] -> Aerodynamic/3(q)
  [theta] -> Body Force/1(theta)
  Body Force/1(Gx) -> Add/1
  Aerodynamic/1(Fx) -> Add/2
  Add1/1 -> Fz/1
  Body Force/2(Gz) -> Add1/1
  Aerodynamic/2(Fz) -> Add1/2
  Demux/7 -> [Ze]
  THR/1 -> Throttle/1(THR)
  Add/1 -> Sum/2
  Sum/1 -> Fx/1
  Throttle/1(Out1) -> Sum/1
  Control System/1 -> [ELE]
  [ELE] -> Aerodynamic/4(del_e)
  Environment/1 -> [rho]

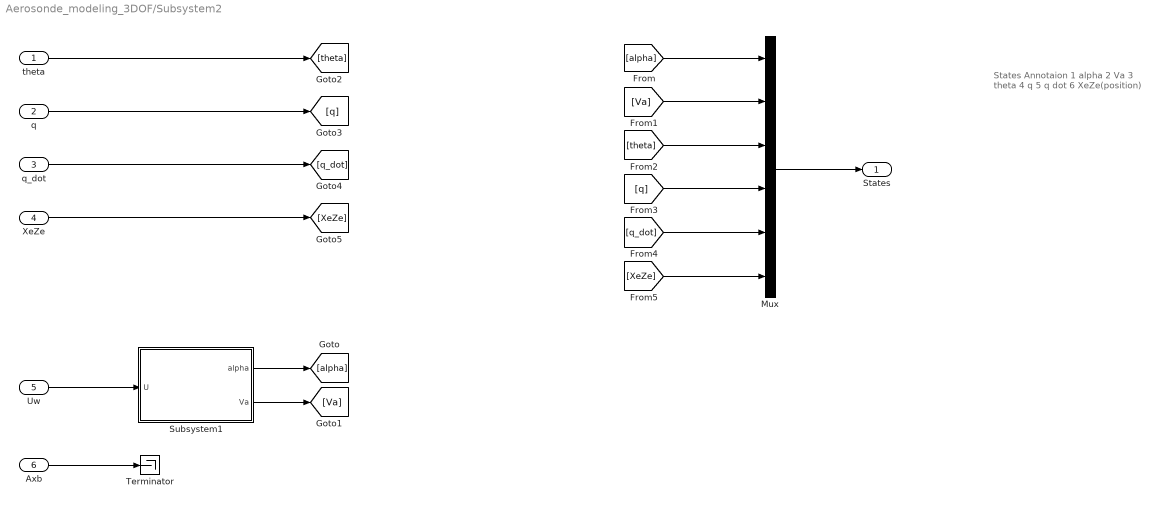
== system Aerosonde_modeling_3DOF/Subsystem2 ==
  note: States Annotaion
      | 1 alpha
      | 2 Va
      | 3 theta
      | 4 q
      | 5 q dot
      | 6 XeZe(position)
  theta : Inport
  q : Inport  Port=2
  q_dot : Inport  Port=3
  XeZe : Inport  Port=4
  Uw : Inport  Port=5
  Axb : Inport  Port=6
  Mux : Mux  Inputs=6
  Subsystem1 : Subsystem
  Terminator : Terminator
  States : Outport
  wires:
  Uw/1 -> Subsystem1/1(U)
  Subsystem1/1(alpha) -> [alpha]
  Subsystem1/2(Va) -> [Va]
  theta/1 -> [theta]
  q/1 -> [q]
  q_dot/1 -> [q_dot]
  XeZe/1 -> [XeZe]
  Axb/1 -> Terminator/1
  [alpha] -> Mux/1
  [Va] -> Mux/2
  [theta] -> Mux/3
  [q] -> Mux/4
  [q_dot] -> Mux/5
  [XeZe] -> Mux/6
  Mux/1 -> States/1

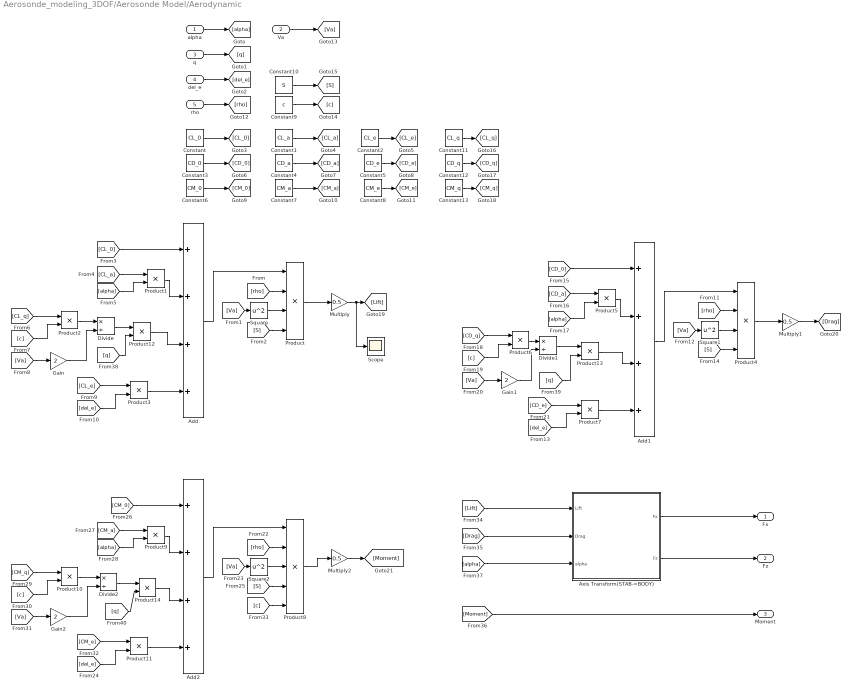
== system Aerosonde_modeling_3DOF/Aerosonde Model/Aerodynamic ==
  alpha : Inport
  Va : Inport  Port=2
  q : Inport  Port=3
  del_e : Inport  Port=4
  rho : Inport  Port=5
  Add : Sum  Inputs=++++
  Add1 : Sum  Inputs=++++
  Add2 : Sum  Inputs=++++
  Axis Transform(STAB->BODY) : Subsystem
  Constant : Constant  Value=CL_0
  Constant1 : Constant  Value=CL_a
  Constant10 : Constant  Value=S
  Constant11 : Constant  Value=CL_q
  Constant12 : Constant  Value=CD_q
  Constant13 : Constant  Value=CM_q
  Constant2 : Constant  Value=CL_e
  Constant3 : Constant  Value=CD_0
  Constant4 : Constant  Value=CD_a
  Constant5 : Constant  Value=CD_e
  Constant6 : Constant  Value=CM_0
  Constant7 : Constant  Value=CM_a
  Constant8 : Constant  Value=CM_e
  Constant9 : Constant  Value=c
  Divide : Product  Inputs=*/
  Divide1 : Product  Inputs=*/
  Divide2 : Product  Inputs=*/
  Gain : Gain  Gain=2
  Gain1 : Gain  Gain=2
  Gain2 : Gain  Gain=2
  Multiply : Gain  Gain=0.5
  Multiply1 : Gain  Gain=0.5
  Multiply2 : Gain  Gain=0.5
  Product : Product  Inputs=4
  Product{1..3,5..7,9..14} (12 alike) : Product
  Product4 : Product  Inputs=4
  Product8 : Product  Inputs=5
  Scope : Scope
  Square : Math  Operator=square
  Square1 : Math  Operator=square
  Square2 : Math  Operator=square
  Fx : Outport
  Fz : Outport  Port=2
  Moment : Outport  Port=3
  wires:
  alpha/1 -> [alpha]
  q/1 -> [q]
  del_e/1 -> [del_e]
  Constant/1 -> [CL_0]
  Constant1/1 -> [CL_a]
  Constant2/1 -> [CL_e]
  Constant3/1 -> [CD_0]
  Constant4/1 -> [CD_a]
  Constant5/1 -> [CD_e]
  Constant6/1 -> [CM_0]
  Constant7/1 -> [CM_a]
  Constant8/1 -> [CM_e]
  rho/1 -> [rho]
  Va/1 -> [Va]
  Constant9/1 -> [c]
  Add/1 -> Product/1
  Multiply/1 -> Scope/1, [Lift]
  Product/1 -> Multiply/1
  [rho] -> Product/2
  [Va] -> Square/1
  Square/1 -> Product/3
  Constant10/1 -> [S]
  [S] -> Product/4
  [CL_0] -> Add/1
  [CL_a] -> Product1/1
  [alpha] -> Product1/2
  Product1/1 -> Add/2
  Constant11/1 -> [CL_q]
  Constant12/1 -> [CD_q]
  Constant13/1 -> [CM_q]
  [c] -> Product2/2
  [CL_q] -> Product2/1
  Product2/1 -> Divide/1
  [Va] -> Gain/1
  Gain/1 -> Divide/2
  Product3/1 -> Add/4
  [CL_e] -> Product3/1
  [del_e] -> Product3/2
  [c] -> Product6/2
  [S] -> Product4/4
  [CD_q] -> Product6/1
  Multiply1/1 -> [Drag]
  [alpha] -> Product5/2
  Product6/1 -> Divide1/1
  [CD_a] -> Product5/1
  [CD_e] -> Product7/1
  [del_e] -> Product7/2
  Product4/1 -> Multiply1/1
  Product7/1 -> Add1/4
  [Va] -> Square1/1
  Product5/1 -> Add1/2
  [Va] -> Gain1/1
  [CD_0] -> Add1/1
  [rho] -> Product4/2
  Gain1/1 -> Divide1/2
  Square1/1 -> Product4/3
  Add1/1 -> Product4/1
  [c] -> Product10/2
  [S] -> Product8/4
  [CM_q] -> Product10/1
  Multiply2/1 -> [Moment]
  [alpha] -> Product9/2
  Product10/1 -> Divide2/1
  [CM_a] -> Product9/1
  [CM_e] -> Product11/1
  [del_e] -> Product11/2
  Product8/1 -> Multiply2/1
  Product11/1 -> Add2/4
  [Va] -> Square2/1
  Product9/1 -> Add2/2
  [Va] -> Gain2/1
  [CM_0] -> Add2/1
  [rho] -> Product8/2
  Gain2/1 -> Divide2/2
  Square2/1 -> Product8/3
  Add2/1 -> Product8/1
  [c] -> Product8/5
  [Lift] -> Axis Transform(STAB->BODY)/1(Lift)
  [Drag] -> Axis Transform(STAB->BODY)/2(Drag)
  Axis Transform(STAB->BODY)/1(Fx) -> Fx/1
  Axis Transform(STAB->BODY)/2(Fz) -> Fz/1
  [Moment] -> Moment/1
  [alpha] -> Axis Transform(STAB->BODY)/3(alpha)
  Divide/1 -> Product12/1
  Product12/1 -> Add/3
  [q] -> Product12/2
  [q] -> Product13/2
  Divide1/1 -> Product13/1
  Product13/1 -> Add1/3
  [q] -> Product14/2
  Divide2/1 -> Product14/1
  Product14/1 -> Add2/3

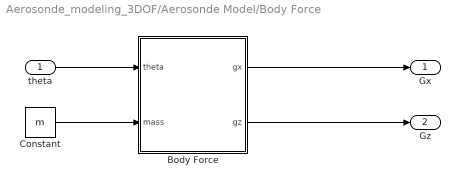
== system Aerosonde_modeling_3DOF/Aerosonde Model/Body Force ==
  theta : Inport
  Body Force : MATLAB Function  TreatAsAtomicUnit=on
  Constant : Constant  Value=m
  Gx : Outport
  Gz : Outport  Port=2
  wires:
  Constant/1 -> Body Force/2(mass)
  theta/1 -> Body Force/1(theta)
  Body Force/1(gx) -> Gx/1
  Body Force/2(gz) -> Gz/1

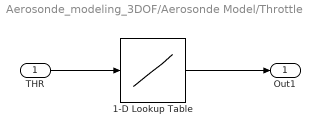
== system Aerosonde_modeling_3DOF/Aerosonde Model/Throttle ==
  THR : Inport
  1-D Lookup Table : Lookup_n-D  NumberOfTableDimensions=1  BreakpointsForDimension1=[0 1]  Table=[0 30]  InternalRulePriority=Speed  RndMeth=Simplest
  Out1 : Outport
  wires:
  THR/1 -> 1-D Lookup Table/1
  1-D Lookup Table/1 -> Out1/1

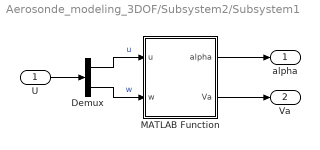
== system Aerosonde_modeling_3DOF/Subsystem2/Subsystem1 ==
  U : Inport
  Demux : Demux  Outputs=2
  MATLAB Function : MATLAB Function  TreatAsAtomicUnit=on
  alpha : Outport
  Va : Outport  Port=2
  wires:
  U/1 -> Demux/1
  Demux/1 -> MATLAB Function/1(u)  "u"
  Demux/2 -> MATLAB Function/2(w)  "w"
  MATLAB Function/1(alpha) -> alpha/1
  MATLAB Function/2(Va) -> Va/1

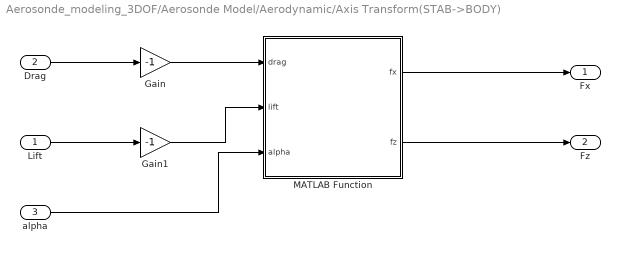
== system Aerosonde_modeling_3DOF/Aerosonde Model/Aerodynamic/Axis Transform(STAB->BODY) ==
  Lift : Inport
  Drag : Inport  Port=2
  alpha : Inport  Port=3
  Gain : Gain  Gain=-1
  Gain1 : Gain  Gain=-1
  MATLAB Function : MATLAB Function  TreatAsAtomicUnit=on
  Fx : Outport
  Fz : Outport  Port=2
  wires:
  Lift/1 -> Gain1/1
  Drag/1 -> Gain/1
  Gain1/1 -> MATLAB Function/2(lift)
  Gain/1 -> MATLAB Function/1(drag)
  MATLAB Function/1(fx) -> Fx/1
  MATLAB Function/2(fz) -> Fz/1
  alpha/1 -> MATLAB Function/3(alpha)

== matlab function Aerosonde_modeling_3DOF/Aerosonde Model/Body Force/Body Force ==
  data: theta input; gx output; gz output; mass input
function [gx, gz] = fcn(theta, mass)

m = mass;
g = 9.84;

gx = -m*g*sin(theta);
gz = m*g*cos(theta);

== matlab function Aerosonde_modeling_3DOF/Subsystem2/Subsystem1/MATLAB Function ==
  data: u input; alpha output; w input; Va output
function [alpha, Va] = fcn(u,w)

% if(u == 0)
%     u = 0.00001;
% end
alpha = atan(w/u);
Va = sqrt(u^2 + w^2);

== matlab function Aerosonde_modeling_3DOF/Aerosonde Model/Aerodynamic/Axis Transform(STAB->BODY)/MATLAB Function ==
  data: drag input; fx output; lift input; fz output; alpha input
function [fx, fz] = STAB2BODY(drag, lift, alpha)

fx = cos(alpha)*drag - sin(alpha)*lift;
fz = sin(alpha)*drag + cos(alpha)*lift;

end
